simulink model "Kalman_Filter_Simulink_Example_adap_SMNSF"  (R2018a)
settings: Solver=FixedStepAuto  StartTime=0.0  StopTime=40  FixedStep=.01  RelTol=1e-3
values from neighbouring files (symbols this model uses):
  g = 9.81    [Kalman_Filter_Simulink_Example_params_EKF.m]
  l = 0.5    [Kalman_Filter_Simulink_Example_params_EKF.m]
  P0 = [10 0; 0 10]    [Kalman_Filter_Simulink_Example_params_EKF.m]
  Q = 1e-4    (= 0.0001)    [Kalman_Filter_Simulink_Example_params_EKF.m]
  Q0 = 2e-4    (= 0.0002)    [Kalman_Filter_Simulink_Example_params_EKF.m]
  R = 1e-3    (= 0.001)    [Kalman_Filter_Simulink_Example_params_EKF.m]
  R0 = 2e-3    (= 0.002)    [Kalman_Filter_Simulink_Example_params_EKF.m]
  theta0 = pi/4    (= 0.785398163397)    [Kalman_Filter_Simulink_Example_params_EKF.m]
  Ts = 0.01    [Kalman_Filter_Simulink_Example_params_EKF.m]
libraries: Bias x9, simulink x4, sharedTrackingLibrary x1, Meldas_Library x1
settings Model: Creator=mulusoy  LastModifiedBy=hussein
settings OptimizationCC: DefaultParameterBehavior=Inlined  PassReuseOutputArgsAs=Individual arguments
settings DebuggingCC: ParameterTunabilityLossMsg=error
settings SFSimCC: MATLABDynamicMemAlloc=off
settings RTWCC: SystemTargetFile=ert.tlc  TemplateMakefile=ert_default_tmf  GenerateReport=on  IncludeHyperlinkInReport=on  LaunchReport=on  GenerateTraceInfo=on  GenerateTraceReport=on  GenerateTraceReportSl=on  GenerateTraceReportSf=on  GenerateTraceReportEml=on  CheckMdlBeforeBuild=Warning
settings CodeAppCC: GenerateComments=off  IgnoreCustomStorageClasses=off  SimulinkBlockComments=off
settings ERTTargetCC: TargetLangStandard=C99 (ISO)  GenerateSampleERTMain=on  InlinedParameterPlacement=NonHierarchical  ERTCustomFileTemplate=example_file_process.tlc
settings SimscapeCC: SimscapeNormalizeSystem=off

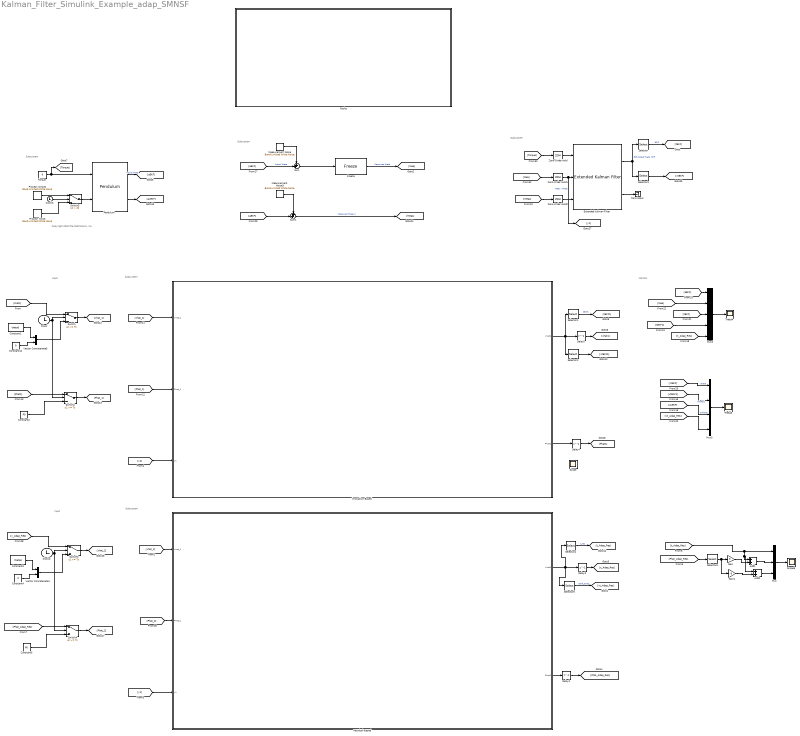
== system Kalman_Filter_Simulink_Example_adap_SMNSF ==
  note: Subsystem
  note: Subsystem
  note: Monitor
  note: Input
  note: Input
  note: Subsystem
  note: Subsystem
  note: Copyright 2018 The MathWorks, Inc.
  note: Subsystem
  Add1 : Sum
  Add2 : Sum
  Clock : Clock
      settings: Decimation=1000
  Clock2 : Clock
      settings: Decimation=1000
  Clock3 : Clock
  Constant1 : Constant  Value=theta0
  Constant12 : Constant  Value=0
  Constant2 : Constant  Value=P0
  Constant3 : Constant  Value=theta0
  Constant4 : Constant  Value=0
  Constant5 : Constant  Value=P0
  Delay{2..5} (4 alike) : Delay  DelayLength=1
  Extended Kalman Filter : sharedTrackingLibrary/Extended Kalman Filter  StateTransitionFcn=myStateTransitionFcn  HasStateTransitionJacobianFcn=off  HasAdditiveProcessNoise=Additive  ProcessNoise=diag([0,Q0])  HasTimeVaryingProcessNoise=off  HasStateTransitionFcnExtraArgument=1  InitialState=[pi/4 0]  InitialStateCovariance=10  MeasurementFcn1=myMeasurementFcn  HasMeasurementJacobianFcn1=off  HasMeasurementEnablePort1=off  HasAdditiveMeasurementNoise1=Additive  MeasurementNoise1=R0  HasTimeVaryingMeasurementNoise1=off  HasMeasurementFcnExtraArgument1=0  MeasurementFcn2=myMeasurementFcn  HasMeasurementJacobianFcn2=off  HasMeasurementEnablePort2=off  HasAdditiveMeasurementNoise2=Additive  MeasurementNoise2=R0  HasTimeVaryingMeasurementNoise2=off  HasMeasurementFcnExtraArgument2=0  MeasurementFcn3=myMeasurementFcn  HasMeasurementJacobianFcn3=off  HasMeasurementEnablePort3=off  HasAdditiveMeasurementNoise3=Additive  MeasurementNoise3=1  HasTimeVaryingMeasurementNoise3=off  HasMeasurementFcnExtraArgument3=0  MeasurementFcn4=myMeasurementFcn  HasMeasurementJacobianFcn4=off  HasMeasurementEnablePort4=off  HasAdditiveMeasurementNoise4=Additive  MeasurementNoise4=1  HasTimeVaryingMeasurementNoise4=off  HasMeasurementFcnExtraArgument4=0  MeasurementFcn5=myMeasurementFcn  HasMeasurementJacobianFcn5=off  HasMeasurementEnablePort5=off  HasAdditiveMeasurementNoise5=Additive  MeasurementNoise5=1  HasTimeVaryingMeasurementNoise5=off  HasMeasurementFcnExtraArgument5=0  EnableMultirate=off  StateTransitionFcnSampleTime=1  MeasurementFcn1SampleTime=1  MeasurementFcn2SampleTime=1  MeasurementFcn3SampleTime=1  MeasurementFcn4SampleTime=1  MeasurementFcn5SampleTime=1  UseCurrentEstimator=on  OutputStateCovariance=on  DataType=double  SampleTime=Ts  NumberOfMeasurements=2
      settings: SourceProductName=Control System Toolbox  SourceProductBaseCode=CT
  Faults : Subsystem
  Freeze : Bias/Freeze  Time=5
  Gain : Gain  Gain=3
  Gain1 : Gain  Gain=-3
  Innovation-Based : Subsystem
  Measurement Noise : simulink/Sources/Band-Limited White Noise  Cov=R*Ts  Ts=Ts  seed=[12347]
  Measurement Noise3 : simulink/Sources/Band-Limited White Noise  Cov=R*Ts  Ts=Ts  seed=[12347]
  Mux : Mux  Inputs=3
  Mux2 : Mux  Inputs=5
  Mux3 : Mux
  Pendulum : Meldas_Library/Pendulum  theta_0=pi/3  theta_dot_0=0
  Process Noise2 : simulink/Sources/Band-Limited White Noise  Cov=Q*Ts*1000  Ts=Ts  seed=[12347]
  Process Noise : simulink/Sources/Band-Limited White Noise  Cov=0  Ts=Ts  seed=[23341]
  Residual-Based : Subsystem
  Scope5 : Scope
  Selector : Selector  InputPortWidth=2  IndexOptions=Index vector (dialog)  Indices=1  OutputSizes=1
  Selector1 : Selector  InputPortWidth=2  IndexOptions=Index vector (dialog)  Indices=1  OutputSizes=1
  Selector2 : Selector  InputPortWidth=2  IndexOptions=Index vector (dialog)  Indices=2  OutputSizes=1
  Selector3 : Selector  InputPortWidth=2  IndexOptions=Index vector (dialog)  Indices=2  OutputSizes=1
  Selector4 : Selector  InputPortWidth=2  IndexOptions=Index vector (dialog)  Indices=1  OutputSizes=1
  Selector5 : Selector  InputPortWidth=2  IndexOptions=Index vector (dialog)  Indices=2  OutputSizes=1
  Selector6 : Selector  NumberOfDimensions=2  InputPortWidth=3  IndexOptions=Index vector (dialog),Index vector (dialog)  Indices=1,1  OutputSizes=1,1
  Sum : Sum  Inputs=++|
  Sum1 : Sum  Inputs=++|
  Switch{,1,3..4} (4 alike) : Switch  Threshold=Ts
  Switch5 : Switch  Criteria=u2 > Threshold  Threshold=40
  Terminator : Terminator
  Theta4 : Scope
  Theta5 : Scope
  Torque : Constant  Value=0
  Vector Concatenate1 : Concatenate
  Vector Concatenate5 : Concatenate
  Zero-Order Hold : ZeroOrderHold  SampleTime=Ts
  Zero-Order Hold1 : ZeroOrderHold  SampleTime=Ts
  Zero-Order Hold2 : ZeroOrderHold  SampleTime=Ts
  Scope : Scope
  wires:
  Clock/1 -> Switch1/2, Switch/2
  Constant1/1 -> Vector Concatenate5/1
  Constant2/1 -> Switch1/3
  Constant12/1 -> Vector Concatenate5/2
  Vector Concatenate5/1 -> Switch/3
  [xhat1] -> Switch/1
  [Phat1] -> Switch1/1
  Switch/1 -> [xhat_1]
  Switch1/1 -> [Phat_1]
  [Phat_1] -> Innovation-Based/2(Phat_1)
  [y1] -> Innovation-Based/3(y1)
  Innovation-Based/2(Phat1) -> Delay4/1
  Selector2/1 -> [vtEKF1]
  Innovation-Based/1(xhat1) -> Selector2/1, Selector1/1, Delay5/1
  Selector1/1 -> [tEKF1]  "tEKF1"
  [xhat_1] -> Innovation-Based/1(xhat_1)
  Residual-Based/2(Phat1) -> Delay2/1
  Residual-Based/1(xhat1) -> Selector5/1, Selector4/1, Delay3/1
  Selector5/1 -> [vt_Adap_Res]  "vEKF_adap"
  [y1] -> Residual-Based/3(y1)
  Clock2/1 -> Switch4/2, Switch3/2
  Switch4/1 -> [Phat_2]
  Constant5/1 -> Switch4/3
  Vector Concatenate1/1 -> Switch3/3
  Constant3/1 -> Vector Concatenate1/1
  Switch3/1 -> [xhat_2]
  [Phat_Adap_Res] -> Switch4/1
  Constant4/1 -> Vector Concatenate1/2
  [x_Adap_Res] -> Switch3/1
  [xhat_2] -> Residual-Based/1(xhat_1)
  [Phat_2] -> Residual-Based/2(Phat_1)
  [Mea] -> Mux2/2
  [vtEKF] -> Mux3/1  "vtheta"
  Mux3/1 -> Theta5/1
  [tEKF1] -> Mux2/4
  Mux2/1 -> Theta4/1
  [vtEKF1] -> Mux3/2  "vtheta1"
  [avEKF] -> Mux3/3  "aVtheta"
  [tEKF] -> Mux2/3
  [aEKF] -> Mux2/1
  [vt_Adap_Res] -> Mux3/4
  [t_Adap_Res] -> Mux2/5
  [Phat_Adap_Res] -> Selector6/1
  [t_Adap_Res] -> Add2/1, Add1/1, Mux/1
  Selector6/1 -> Gain1/1, Gain/1
  Gain/1 -> Add1/2
  Add1/1 -> Mux/2
  Gain1/1 -> Add2/2
  Add2/1 -> Mux/3
  Mux/1 -> Scope5/1
  Selector4/1 -> [t_Adap_Res]  "t_res"
  Delay2/1 -> [Phat_Adap_Res]
  Delay3/1 -> [x_Adap_Res]
  Delay4/1 -> [Phat1]
  Delay5/1 -> [xhat1]
  Pendulum/1 -> [aEKF]  "Actual theta"
  Pendulum/2 -> [avEKF]
  [aEKF] -> Sum1/2
  Sum/1 -> Freeze/1
  Process Noise/1 -> Switch5/3
  Measurement Noise/1 -> Sum/1
  [aEKF] -> Sum/2  "Actual theta"
  Clock3/1 -> Switch5/2
  Torque/1 -> Pendulum/1, [Torque]
  Measurement Noise3/1 -> Sum1/1
  Freeze/1 -> [Mea]  "Measured theta"
  Process Noise2/1 -> Switch5/1
  Sum1/1 -> [Mea1]  "Measured theta 2"
  Switch5/1 -> Pendulum/2
  Zero-Order Hold1/1 -> [y1], Extended Kalman Filter/2  "Meas  Theta"
  Extended Kalman Filter/1 -> Selector3/1, Selector/1  "Estimated theta  EKF"
  Zero-Order Hold/1 -> Extended Kalman Filter/1
  Selector/1 -> [tEKF]  "tEKF"
  Selector3/1 -> [vtEKF]
  [Mea] -> Zero-Order Hold1/1
  [Mea1] -> Zero-Order Hold2/1
  Zero-Order Hold2/1 -> Extended Kalman Filter/3
  [Torque] -> Zero-Order Hold/1
  Extended Kalman Filter/2 -> Terminator/1

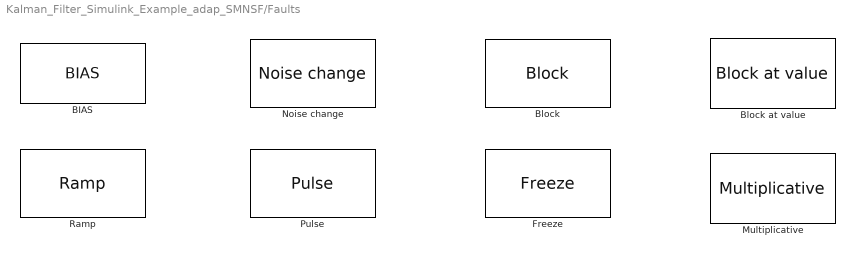
== system Kalman_Filter_Simulink_Example_adap_SMNSF/Faults ==
  BIAS : Bias/BIAS  Bias=0  Time=0
  Block : Bias/Block  Noise=0  Time=0
  Block at value : Bias/Block at value  Value=0  Time=0
  Freeze : Bias/Freeze  Time=0
  Multiplicative : Bias/Multiplicative  Gain=0  Time=0
  Noise change : Bias/Noise change  Noise_add=0  Time=0
  Pulse : Bias/Pulse  Pulse_value=0.1  Pulse_periode=0  Pulse_width=0  Time=0
  Ramp : Bias/Ramp  Slope=0  Time=0

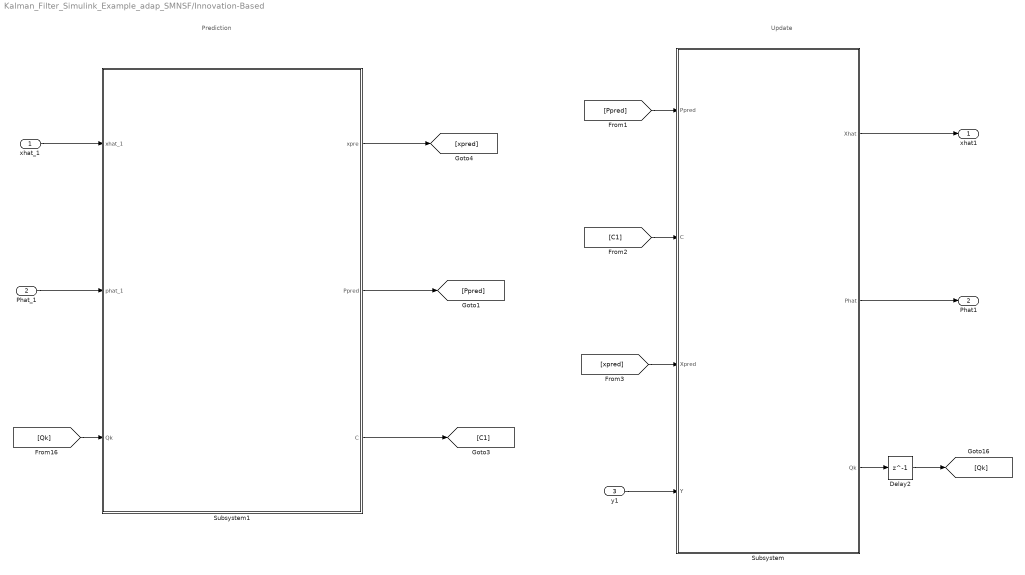
== system Kalman_Filter_Simulink_Example_adap_SMNSF/Innovation-Based ==
  note: Update
  note: Prediction
  xhat_1 : Inport
  Phat_1 : Inport  Port=2
  y1 : Inport  Port=3
  Delay2 : Delay  DelayLength=1  SampleTime=Ts
  Subsystem : Subsystem
  Subsystem1 : Subsystem
  xhat1 : Outport
  Phat1 : Outport  Port=2
  wires:
  [Ppred] -> Subsystem/1(Ppred)
  Subsystem/3(Qk) -> Delay2/1
  y1/1 -> Subsystem/4("Y ")
  Delay2/1 -> [Qk]
  Subsystem/2("Phat ") -> Phat1/1
  Subsystem1/1(xpre) -> [xpred]
  [C1] -> Subsystem/2(C)
  Phat_1/1 -> Subsystem1/2("phat_1 ")
  [xpred] -> Subsystem/3(Xpred)
  xhat_1/1 -> Subsystem1/1(xhat_1)
  Subsystem1/2(Ppred) -> [Ppred]
  Subsystem1/3("C ") -> [C1]
  Subsystem/1(Xhat) -> xhat1/1
  [Qk] -> Subsystem1/3("Qk ")

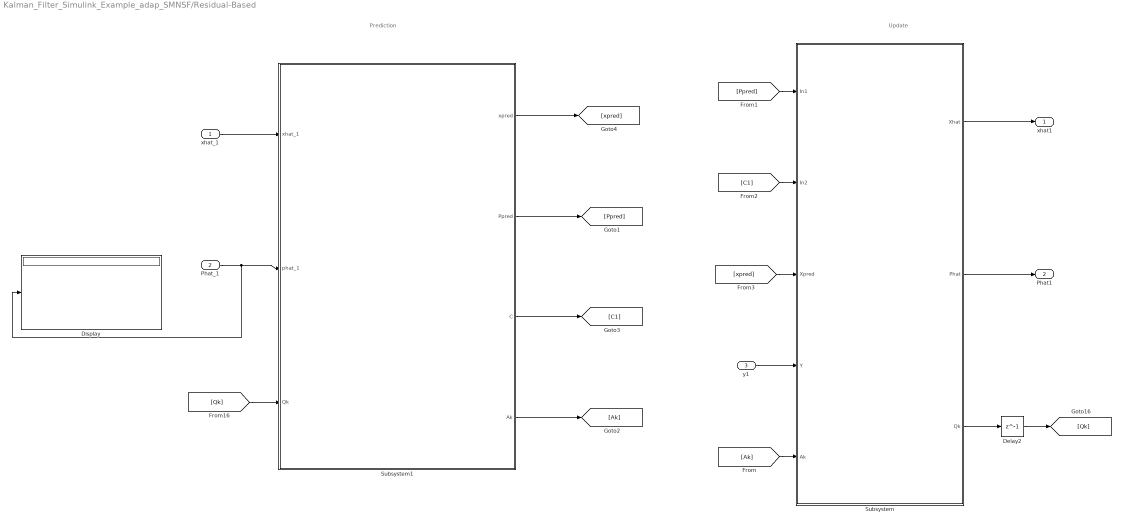
== system Kalman_Filter_Simulink_Example_adap_SMNSF/Residual-Based ==
  note: Update
  note: Prediction
  xhat_1 : Inport
  Phat_1 : Inport  Port=2
  y1 : Inport  Port=3
  Delay2 : Delay  DelayLength=1  SampleTime=Ts
  Display : Display
  Subsystem : Subsystem
  Subsystem1 : Subsystem
  xhat1 : Outport
  Phat1 : Outport  Port=2
  wires:
  [Ppred] -> Subsystem/1(In1)
  y1/1 -> Subsystem/4("Y ")
  Delay2/1 -> [Qk]
  Subsystem/2("Phat ") -> Phat1/1
  Subsystem1/1(xpred) -> [xpred]
  [C1] -> Subsystem/2(In2)
  Phat_1/1 -> Display/1, Subsystem1/2(phat_1)
  [xpred] -> Subsystem/3(Xpred)
  xhat_1/1 -> Subsystem1/1(xhat_1)
  Subsystem1/2(Ppred) -> [Ppred]
  Subsystem1/3("C ") -> [C1]
  Subsystem/1(Xhat) -> xhat1/1
  [Qk] -> Subsystem1/3("Qk ")
  Subsystem1/4(Ak) -> [Ak]
  [Ak] -> Subsystem/5("Ak ")
  Subsystem/3(Qk) -> Delay2/1

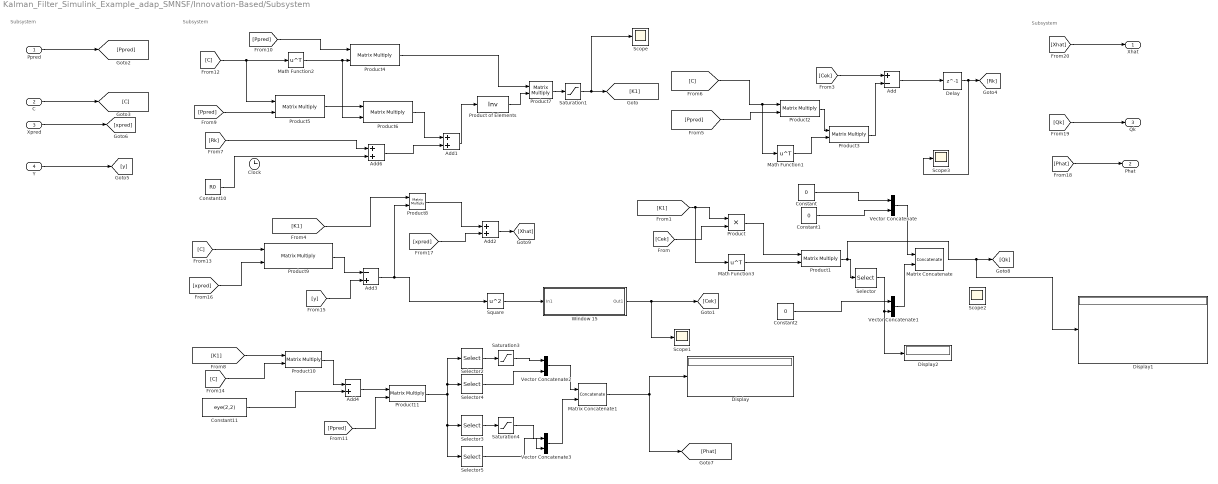
== system Kalman_Filter_Simulink_Example_adap_SMNSF/Innovation-Based/Subsystem ==
  note: Subsystem
  note: Subsystem
  note: Subsystem
  Ppred : Inport
  C : Inport  Port=2
  Xpred : Inport  Port=3
  "Y " : Inport  Port=4
  Add : Sum  Inputs=+-
  Add1 : Sum
  Add2 : Sum
  Add3 : Sum  Inputs=-+
  Add4 : Sum  Inputs=-+
  Add6 : Sum
  Clock : Clock
  Constant : Constant  Value=0
  Constant1 : Constant  Value=0
  Constant10 : Constant  Value=R0
  Constant11 : Constant  Value=eye(2,2)
  Constant2 : Constant  Value=0
  Delay : Delay  DelayLength=1
  Display : Display
  Display1 : Display
  Display2 : Display
  Math Function1 : Math  Operator=transpose  SaturateOnIntegerOverflow=on
  Math Function2 : Math  Operator=transpose  SaturateOnIntegerOverflow=on
  Math Function3 : Math  Operator=transpose  SaturateOnIntegerOverflow=on
  Matrix Concatenate : Concatenate  Mode=Multidimensional array  ConcatenateDimension=2
  Matrix Concatenate1 : Concatenate  Mode=Multidimensional array  ConcatenateDimension=2
  Product : Product
  Product of Elements : Product  Inputs=/  Multiplication=Matrix(*)
  Product{1..11} (11 alike) : Product  Multiplication=Matrix(*)
  Saturation1 : Saturate  UpperLimit=1  LowerLimit=0
  Saturation3 : Saturate  UpperLimit=1  LowerLimit=0
  Saturation4 : Saturate  UpperLimit=1  LowerLimit=0
  Scope{,1..3} (4 alike) : Scope
  Selector : Selector  NumberOfDimensions=2  InputPortWidth=3  IndexOptions=Index vector (dialog),Index vector (dialog)  Indices=2,2  OutputSizes=1,1
  Selector2 : Selector  NumberOfDimensions=2  InputPortWidth=3  IndexOptions=Index vector (dialog),Index vector (dialog)  Indices=1,1  OutputSizes=1,1
  Selector3 : Selector  NumberOfDimensions=2  InputPortWidth=3  IndexOptions=Index vector (dialog),Index vector (dialog)  Indices=2,2  OutputSizes=1,1
  Selector4 : Selector  NumberOfDimensions=2  InputPortWidth=3  IndexOptions=Index vector (dialog),Index vector (dialog)  Indices=2,1  OutputSizes=1,1
  Selector5 : Selector  NumberOfDimensions=2  InputPortWidth=3  IndexOptions=Index vector (dialog),Index vector (dialog)  Indices=1,2  OutputSizes=1,1
  Square : Math  Operator=square  SaturateOnIntegerOverflow=on
  Vector Concatenate{,1..3} (4 alike) : Concatenate
  Window 15 : Subsystem
  Xhat : Outport  PortDimensions=[2,1]
  "Phat " : Outport  Port=2  PortDimensions=[2,2]
  Qk : Outport  Port=3  PortDimensions=[2,2]
  wires:
  Ppred/1 -> [Ppred]
  C/1 -> [C]
  Xpred/1 -> [xpred]
  "Y "/1 -> [y]
  [Xhat] -> Xhat/1
  [Phat] -> "Phat "/1
  [Qk] -> Qk/1
  Product2/1 -> Product3/1
  [xpred] -> Add2/2
  Add4/1 -> Product11/1
  [Ppred] -> Product2/2
  [K1] -> Product10/1
  [xpred] -> Product9/2
  [K1] -> Product8/1
  Math Function1/1 -> Product3/2
  Square/1 -> Window 15/1(In1)
  [K1] -> Math Function3/1, Product/1
  [Cek] -> Add/1
  [Cek] -> Product/2
  Math Function2/1 -> Product6/2, Product4/2
  Product of Elements/1 -> Product7/2
  Add1/1 -> Product of Elements/1
  Product8/1 -> Add2/1
  Product3/1 -> Add/2
  Product/1 -> Product1/1
  [Rk] -> Add6/1
  Constant11/1 -> Add4/2
  [Ppred] -> Product11/2
  [y] -> Add3/2
  [C] -> Math Function1/1, Product2/1
  Product10/1 -> Add4/1
  Product6/1 -> Add1/1
  [C] -> Product9/1
  Add3/1 -> Square/1, Product8/2
  Add2/1 -> [Xhat]
  Product4/1 -> Product7/1
  Product5/1 -> Product6/1
  [C] -> Product10/2
  [Ppred] -> Product4/1
  Product9/1 -> Add3/1
  [Ppred] -> Product5/2
  [C] -> Product5/1, Math Function2/1
  Product1/1 -> Display1/1, [Qk], Selector/1
  Constant/1 -> Vector Concatenate/1
  Constant1/1 -> Vector Concatenate/2
  Constant2/1 -> Vector Concatenate1/1
  Vector Concatenate/1 -> Matrix Concatenate/1
  Math Function3/1 -> Product1/2
  Window 15/1(Out1) -> Scope1/1, [Cek]
  Add/1 -> Delay/1
  Vector Concatenate1/1 -> Matrix Concatenate/2
  Selector/1 -> Display2/1, Vector Concatenate1/2
  Constant10/1 -> Add6/2
  Add6/1 -> Add1/2
  Product7/1 -> Saturation1/1
  Delay/1 -> Scope3/1, [Rk]
  Saturation1/1 -> Scope/1, [K1]
  Vector Concatenate2/1 -> Matrix Concatenate1/1
  Matrix Concatenate1/1 -> Display/1, [Phat]
  Selector4/1 -> Vector Concatenate2/2
  Vector Concatenate3/1 -> Matrix Concatenate1/2
  Selector3/1 -> Saturation4/1
  Selector5/1 -> Vector Concatenate3/1
  Saturation3/1 -> Vector Concatenate2/1
  Product11/1 -> Selector5/1, Selector3/1, Selector4/1, Selector2/1
  Saturation4/1 -> Vector Concatenate3/2
  Selector2/1 -> Saturation3/1

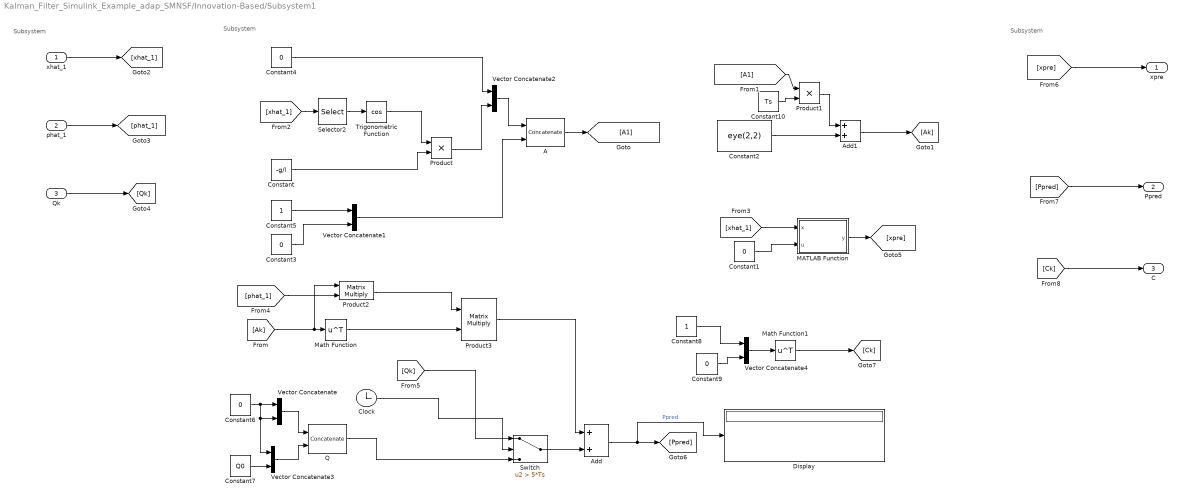
== system Kalman_Filter_Simulink_Example_adap_SMNSF/Innovation-Based/Subsystem1 ==
  note: Subsystem
  note: Subsystem
  note: Subsystem
  xhat_1 : Inport
  "phat_1 " : Inport  Port=2
  "Qk " : Inport  Port=3
  A : Concatenate  Mode=Multidimensional array  ConcatenateDimension=2
  Add : Sum
  Add1 : Sum
  Clock : Clock
      settings: Decimation=1000
  Constant : Constant  Value=-g/l
  Constant{1,3..4,6,9} (5 alike) : Constant  Value=0
  Constant10 : Constant  Value=Ts
  Constant2 : Constant  Value=eye(2,2)
  Constant5 : Constant
  Constant7 : Constant  Value=Q0
  Constant8 : Constant
  Display : Display
  MATLAB Function : MATLAB Function  TreatAsAtomicUnit=on
  Math Function : Math  Operator=transpose  SaturateOnIntegerOverflow=on
  Math Function1 : Math  Operator=transpose  SaturateOnIntegerOverflow=on
  Product : Product
  Product1 : Product
  Product2 : Product  Multiplication=Matrix(*)
  Product3 : Product  Multiplication=Matrix(*)
  Q : Concatenate  Mode=Multidimensional array  ConcatenateDimension=2
  Selector2 : Selector  InputPortWidth=2  IndexOptions=Index vector (dialog)  Indices=1  OutputSizes=1
  Switch : Switch  Criteria=u2 > Threshold  Threshold=5*Ts
  Trigonometric Function : Trigonometry  Operator=cos
  Vector Concatenate{,1..4} (5 alike) : Concatenate
  xpre : Outport
  Ppred : Outport  Port=2
  "C " : Outport  Port=3
  wires:
  "Qk "/1 -> [Qk]
  xhat_1/1 -> [xhat_1]
  "phat_1 "/1 -> [phat_1]
  [xpre] -> xpre/1
  [Ppred] -> Ppred/1
  [Ck] -> "C "/1
  Constant10/1 -> Product1/2
  [A1] -> Product1/1
  Constant/1 -> Product/2
  [xhat_1] -> MATLAB Function/1(x)
  Selector2/1 -> Trigonometric Function/1
  Constant9/1 -> Vector Concatenate4/2
  Vector Concatenate2/1 -> A/1
  Product/1 -> Vector Concatenate2/2
  Constant5/1 -> Vector Concatenate1/1
  A/1 -> [A1]
  Vector Concatenate1/1 -> A/2
  Math Function/1 -> Product3/2
  Product3/1 -> Add/1
  Constant3/1 -> Vector Concatenate1/2
  Product2/1 -> Product3/1
  Vector Concatenate4/1 -> Math Function1/1
  Product1/1 -> Add1/1
  Constant1/1 -> MATLAB Function/2(u)
  Constant7/1 -> Vector Concatenate3/2
  Vector Concatenate3/1 -> Q/2
  [Ak] -> Math Function/1, Product2/1
  Constant8/1 -> Vector Concatenate4/1
  Trigonometric Function/1 -> Product/1
  Add/1 -> Display/1, [Ppred]  "Ppred"
  [xhat_1] -> Selector2/1
  Constant2/1 -> Add1/2
  [phat_1] -> Product2/2
  MATLAB Function/1(y) -> [xpre]
  Clock/1 -> Switch/2
  Add1/1 -> [Ak]
  Math Function1/1 -> [Ck]
  Vector Concatenate/1 -> Q/1
  Constant4/1 -> Vector Concatenate2/1
  Q/1 -> Switch/3
  Constant6/1 -> Vector Concatenate3/1, Vector Concatenate/2, Vector Concatenate/1
  Switch/1 -> Add/2
  [Qk] -> Switch/1

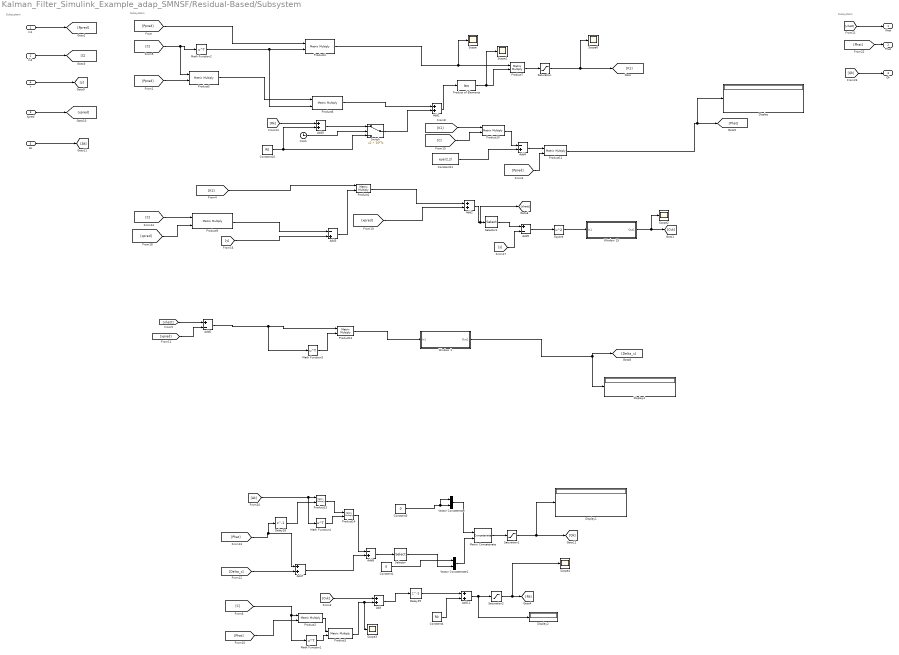
== system Kalman_Filter_Simulink_Example_adap_SMNSF/Residual-Based/Subsystem ==
  note: Subsystem
  note: Subsystem
  note: Subsystem
  In1 : Inport
  In2 : Inport  Port=2
  Xpred : Inport  Port=3
  "Y " : Inport  Port=4
  "Ak " : Inport  Port=5
  Add{,1..2,7,9,11} (6 alike) : Sum
  Add3 : Sum  Inputs=-+
  Add4 : Sum  Inputs=-+
  Add5 : Sum  Inputs=+-
  Add6 : Sum  Inputs=+-
  Add8 : Sum  Inputs=-+
  Clock : Clock
  Constant1 : Constant  Value=0
  Constant10 : Constant  Value=R0
  Constant11 : Constant  Value=eye(2,2)
  Constant3 : Constant  Value=0
  Constant4 : Constant  Value=R0
  Delay28 : Delay  DelayLength=1
  Delay29 : Delay  DelayLength=1
  Display{,1..2,4} (4 alike) : Display
  Math Function{1..4} (4 alike) : Math  Operator=transpose  SaturateOnIntegerOverflow=on
  Matrix Concatenate : Concatenate  Mode=Multidimensional array  ConcatenateDimension=2
  Product of Elements : Product  Inputs=/  Multiplication=Matrix(*)
  Product{1..7,9..14} (13 alike) : Product  Multiplication=Matrix(*)
  Saturation : Saturate  UpperLimit=1  LowerLimit=0
  Saturation1 : Saturate  UpperLimit=1  LowerLimit=0
  Saturation2 : Saturate  UpperLimit=1  LowerLimit=0
  Scope{,1..4,6} (6 alike) : Scope
  Selector : Selector  NumberOfDimensions=2  InputPortWidth=3  IndexOptions=Index vector (dialog),Index vector (dialog)  Indices=2,2  OutputSizes=1,1
  Selector1 : Selector  InputPortWidth=2  IndexOptions=Index vector (dialog)  Indices=1  OutputSizes=1
  Square : Math  Operator=square  SaturateOnIntegerOverflow=on
  Switch : Switch  Criteria=u2 > Threshold  Threshold=20*Ts
  Vector Concatenate : Concatenate
  Vector Concatenate1 : Concatenate
  Window 1 : Subsystem
  Window 15 : Subsystem
  Xhat : Outport  PortDimensions=[2,1]
  "Phat " : Outport  Port=2
  Qk : Outport  Port=3  PortDimensions=[2,2]
  wires:
  Add2/1 -> [xhatt], Selector1/1
  Add5/1 -> Square/1
  [K1] -> Product1/1
  [Ppred] -> Product4/1
  Add3/1 -> Product1/2
  Product of Elements/1 -> Scope1/1, Product7/2
  Product5/1 -> Product6/1
  Product9/1 -> Add3/1
  Math Function2/1 -> Product6/2, Product4/2
  [xhatt] -> Add6/1
  Add1/1 -> Product of Elements/1
  Window 1/1(Out1) -> [Delta_x], Display4/1
  [xpred] -> Add6/2
  Math Function3/1 -> Product12/2
  Product6/1 -> Add1/1
  Selector1/1 -> Add5/1
  Product1/1 -> Add2/1
  [Ppred] -> Product5/2
  Add6/1 -> Product12/1, Math Function3/1
  [C] -> Product9/1
  Window 15/1(Out1) -> Scope2/1, [Cvk]
  [C] -> Product5/1, Math Function2/1
  [y] -> Add3/2
  [y] -> Add5/2
  [xpred] -> Product9/2
  [xpred] -> Add2/2
  "Y "/1 -> [y]
  In1/1 -> [Ppred]
  In2/1 -> [C]
  "Ak "/1 -> [Ak]
  Xpred/1 -> [xpred]
  [xhatt] -> Xhat/1
  [Phat] -> "Phat "/1
  [Qk] -> Qk/1
  Add4/1 -> Product11/1
  [C] -> Product10/2
  Product10/1 -> Add4/1
  [Ppred] -> Product11/2
  [K1] -> Product10/1
  Constant11/1 -> Add4/2
  [Delta_x] -> Add7/2
  [Cvk] -> Add/1
  Math Function1/1 -> Product3/2
  Product13/1 -> Product14/1
  [C] -> Math Function1/1, Product2/1
  Product14/1 -> Add8/1
  Product2/1 -> Product3/1
  [Phat] -> Delay28/1, Add7/1
  Math Function4/1 -> Product14/2
  Add7/1 -> Add8/2
  Product3/1 -> Add/2, Scope3/1
  Vector Concatenate1/1 -> Matrix Concatenate/2
  Constant1/1 -> Vector Concatenate1/1
  Vector Concatenate/1 -> Matrix Concatenate/1
  Constant3/1 -> Vector Concatenate/1, Vector Concatenate/2
  Add8/1 -> Selector/1
  Delay28/1 -> Product13/2
  Add/1 -> Delay29/1
  Product4/1 -> Scope/1, Product7/1
  Product7/1 -> Saturation/1
  [Phat] -> Product2/2
  Delay29/1 -> Add11/1
  Constant4/1 -> Add11/2
  Add11/1 -> Display2/1, Saturation2/1
  Matrix Concatenate/1 -> Saturation1/1
  Selector/1 -> Vector Concatenate1/2
  [Ak] -> Math Function4/1, Product13/1
  Saturation/1 -> Scope6/1, [K1]
  Square/1 -> Window 15/1(In1)
  Switch/1 -> Add1/2
  [Rk] -> Add9/1
  Clock/1 -> Switch/2
  Constant10/1 -> Add9/2, Switch/3
  Saturation1/1 -> [Qk], Display1/1
  Saturation2/1 -> Scope4/1, [Rk]
  Product11/1 -> Display/1, [Phat]
  Product12/1 -> Window 1/1(In1)
  Add9/1 -> Switch/1

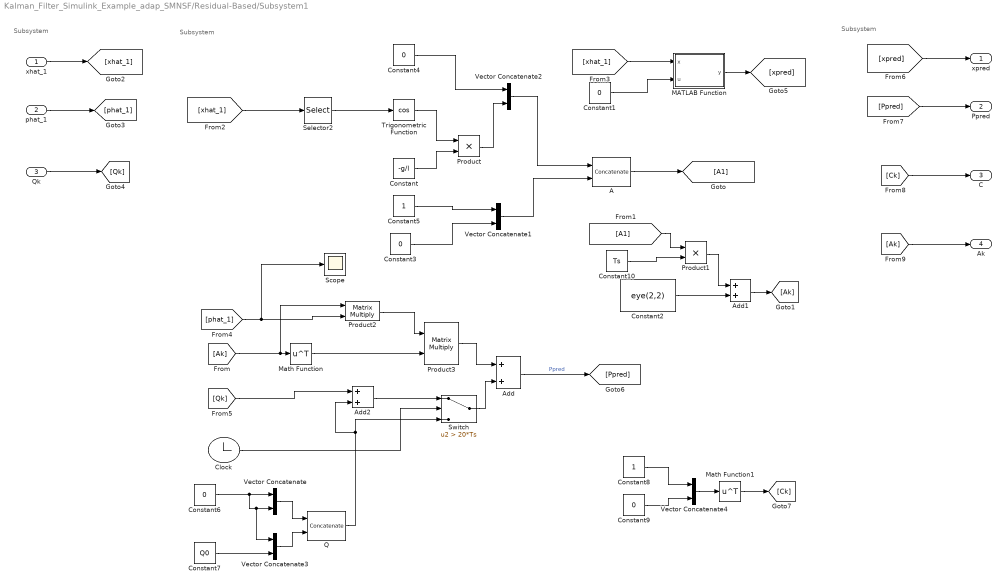
== system Kalman_Filter_Simulink_Example_adap_SMNSF/Residual-Based/Subsystem1 ==
  note: Subsystem
  note: Subsystem
  note: Subsystem
  xhat_1 : Inport
  phat_1 : Inport  Port=2
  "Qk " : Inport  Port=3
  A : Concatenate  Mode=Multidimensional array  ConcatenateDimension=2
  Add : Sum
  Add1 : Sum
  Add2 : Sum
  Clock : Clock
      settings: Decimation=1000
  Constant : Constant  Value=-g/l
  Constant{1,3..4,6,9} (5 alike) : Constant  Value=0
  Constant10 : Constant  Value=Ts
  Constant2 : Constant  Value=eye(2,2)
  Constant5 : Constant
  Constant7 : Constant  Value=Q0
  Constant8 : Constant
  MATLAB Function : MATLAB Function  TreatAsAtomicUnit=on
  Math Function : Math  Operator=transpose  SaturateOnIntegerOverflow=on
  Math Function1 : Math  Operator=transpose  SaturateOnIntegerOverflow=on
  Product : Product
  Product1 : Product
  Product2 : Product  Multiplication=Matrix(*)
  Product3 : Product  Multiplication=Matrix(*)
  Q : Concatenate  Mode=Multidimensional array  ConcatenateDimension=2
  Scope : Scope
  Selector2 : Selector  InputPortWidth=2  IndexOptions=Index vector (dialog)  Indices=1  OutputSizes=1
  Switch : Switch  Criteria=u2 > Threshold  Threshold=20*Ts
  Trigonometric Function : Trigonometry  Operator=cos
  Vector Concatenate{,1..4} (5 alike) : Concatenate
  xpred : Outport
  Ppred : Outport  Port=2
  "C " : Outport  Port=3
  Ak : Outport  Port=4
  wires:
  phat_1/1 -> [phat_1]
  xhat_1/1 -> [xhat_1]
  "Qk "/1 -> [Qk]
  [xpred] -> xpred/1
  [Ppred] -> Ppred/1
  [Ck] -> "C "/1
  [Ak] -> Ak/1
  Add1/1 -> [Ak]
  Constant2/1 -> Add1/2
  [A1] -> Product1/1
  [xhat_1] -> Selector2/1
  A/1 -> [A1]
  Constant4/1 -> Vector Concatenate2/1
  Constant9/1 -> Vector Concatenate4/2
  Vector Concatenate2/1 -> A/1
  Vector Concatenate4/1 -> Math Function1/1
  Trigonometric Function/1 -> Product/1
  [phat_1] -> Scope/1, Product2/2
  Product2/1 -> Product3/1
  Constant10/1 -> Product1/2
  [Ak] -> Product2/1, Math Function/1
  Product/1 -> Vector Concatenate2/2
  Selector2/1 -> Trigonometric Function/1
  Vector Concatenate3/1 -> Q/2
  Vector Concatenate1/1 -> A/2
  Product1/1 -> Add1/1
  Math Function/1 -> Product3/2
  Vector Concatenate/1 -> Q/1
  Constant6/1 -> Vector Concatenate3/1, Vector Concatenate/2, Vector Concatenate/1
  Constant1/1 -> MATLAB Function/2(u)
  Constant5/1 -> Vector Concatenate1/1
  Constant3/1 -> Vector Concatenate1/2
  Constant/1 -> Product/2
  Math Function1/1 -> [Ck]
  Product3/1 -> Add/1
  MATLAB Function/1(y) -> [xpred]
  [xhat_1] -> MATLAB Function/1(x)
  Constant8/1 -> Vector Concatenate4/1
  Constant7/1 -> Vector Concatenate3/2
  Add/1 -> [Ppred]  "Ppred"
  Clock/1 -> Switch/2
  Switch/1 -> Add/2
  [Qk] -> Add2/1
  Q/1 -> Add2/2, Switch/3
  Add2/1 -> Switch/1

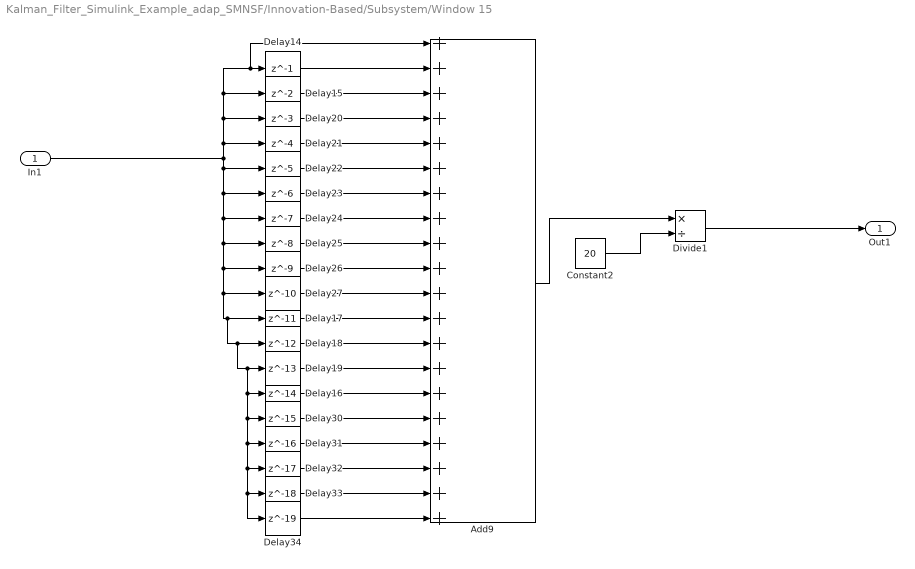
== system Kalman_Filter_Simulink_Example_adap_SMNSF/Innovation-Based/Subsystem/Window 15 ==
  In1 : Inport
  Add9 : Sum  Inputs=20
  Constant2 : Constant  Value=20
  Delay14 : Delay  DelayLength=1  SampleTime=Ts
  Delay15 : Delay  SampleTime=Ts
  Delay16 : Delay  DelayLength=14  SampleTime=Ts
  Delay17 : Delay  DelayLength=11  SampleTime=Ts
  Delay18 : Delay  DelayLength=12  SampleTime=Ts
  Delay19 : Delay  DelayLength=13  SampleTime=Ts
  Delay20 : Delay  DelayLength=3  SampleTime=Ts
  Delay21 : Delay  DelayLength=4  SampleTime=Ts
  Delay22 : Delay  DelayLength=5  SampleTime=Ts
  Delay23 : Delay  DelayLength=6  SampleTime=Ts
  Delay24 : Delay  DelayLength=7  SampleTime=Ts
  Delay25 : Delay  DelayLength=8  SampleTime=Ts
  Delay26 : Delay  DelayLength=9  SampleTime=Ts
  Delay27 : Delay  DelayLength=10  SampleTime=Ts
  Delay30 : Delay  DelayLength=15  SampleTime=Ts
  Delay31 : Delay  DelayLength=16  SampleTime=Ts
  Delay32 : Delay  DelayLength=17  SampleTime=Ts
  Delay33 : Delay  DelayLength=18  SampleTime=Ts
  Delay34 : Delay  DelayLength=19  SampleTime=Ts
  Divide1 : Product  Inputs=*/
  Out1 : Outport
  wires:
  Delay31/1 -> Add9/17
  Delay30/1 -> Add9/16
  Delay14/1 -> Add9/2
  Add9/1 -> Divide1/1
  Delay17/1 -> Add9/12
  Delay19/1 -> Add9/14
  Delay23/1 -> Add9/7
  Delay25/1 -> Add9/9
  Delay26/1 -> Add9/10
  Delay18/1 -> Add9/13
  Delay24/1 -> Add9/8
  Delay20/1 -> Add9/4
  Delay21/1 -> Add9/5
  Delay15/1 -> Add9/3
  Delay32/1 -> Add9/18
  Delay34/1 -> Add9/20
  Delay33/1 -> Add9/19
  Delay22/1 -> Add9/6
  Constant2/1 -> Divide1/2
  Delay27/1 -> Add9/11
  In1/1 -> Delay14/1, Add9/1, Delay15/1, Delay20/1, Delay21/1, Delay34/1, Delay33/1, Delay32/1, Delay31/1, Delay30/1, Delay16/1, Delay19/1, Delay18/1, Delay17/1, Delay27/1, Delay26/1, Delay25/1, Delay24/1, Delay23/1, Delay22/1
  Delay16/1 -> Add9/15
  Divide1/1 -> Out1/1

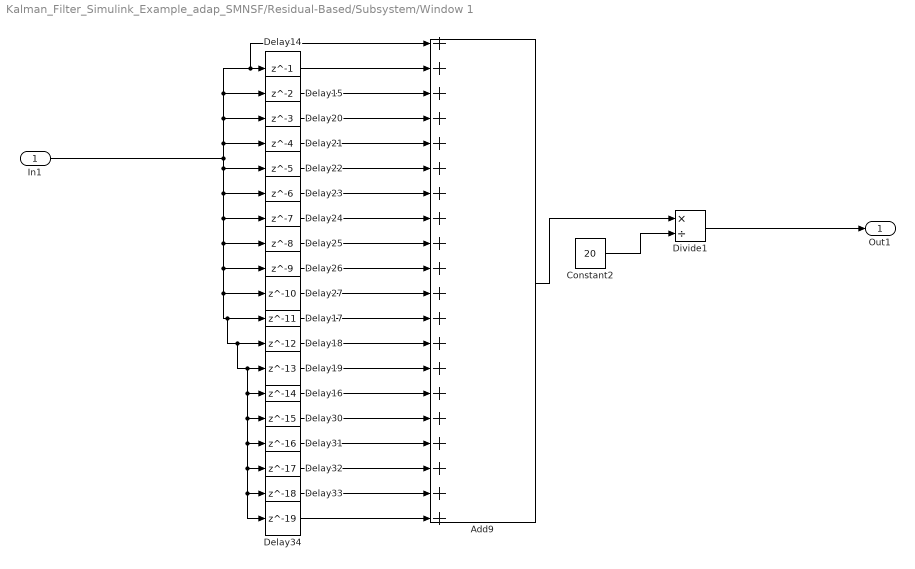
== system Kalman_Filter_Simulink_Example_adap_SMNSF/Residual-Based/Subsystem/Window 1 ==
  In1 : Inport
  Add9 : Sum  Inputs=20
  Constant2 : Constant  Value=20
  Delay14 : Delay  DelayLength=1  SampleTime=Ts
  Delay15 : Delay  SampleTime=Ts
  Delay16 : Delay  DelayLength=14  SampleTime=Ts
  Delay17 : Delay  DelayLength=11  SampleTime=Ts
  Delay18 : Delay  DelayLength=12  SampleTime=Ts
  Delay19 : Delay  DelayLength=13  SampleTime=Ts
  Delay20 : Delay  DelayLength=3  SampleTime=Ts
  Delay21 : Delay  DelayLength=4  SampleTime=Ts
  Delay22 : Delay  DelayLength=5  SampleTime=Ts
  Delay23 : Delay  DelayLength=6  SampleTime=Ts
  Delay24 : Delay  DelayLength=7  SampleTime=Ts
  Delay25 : Delay  DelayLength=8  SampleTime=Ts
  Delay26 : Delay  DelayLength=9  SampleTime=Ts
  Delay27 : Delay  DelayLength=10  SampleTime=Ts
  Delay30 : Delay  DelayLength=15  SampleTime=Ts
  Delay31 : Delay  DelayLength=16  SampleTime=Ts
  Delay32 : Delay  DelayLength=17  SampleTime=Ts
  Delay33 : Delay  DelayLength=18  SampleTime=Ts
  Delay34 : Delay  DelayLength=19  SampleTime=Ts
  Divide1 : Product  Inputs=*/
  Out1 : Outport
  wires:
  Delay31/1 -> Add9/17
  Delay30/1 -> Add9/16
  Delay14/1 -> Add9/2
  Add9/1 -> Divide1/1
  Delay17/1 -> Add9/12
  Delay19/1 -> Add9/14
  Delay23/1 -> Add9/7
  Delay25/1 -> Add9/9
  Delay26/1 -> Add9/10
  Delay18/1 -> Add9/13
  Delay24/1 -> Add9/8
  Delay20/1 -> Add9/4
  Delay21/1 -> Add9/5
  Delay15/1 -> Add9/3
  Delay32/1 -> Add9/18
  Delay34/1 -> Add9/20
  Delay33/1 -> Add9/19
  Delay22/1 -> Add9/6
  Constant2/1 -> Divide1/2
  Delay27/1 -> Add9/11
  In1/1 -> Delay14/1, Add9/1, Delay15/1, Delay20/1, Delay21/1, Delay34/1, Delay33/1, Delay32/1, Delay31/1, Delay30/1, Delay16/1, Delay19/1, Delay18/1, Delay17/1, Delay27/1, Delay26/1, Delay25/1, Delay24/1, Delay23/1, Delay22/1
  Delay16/1 -> Add9/15
  Divide1/1 -> Out1/1

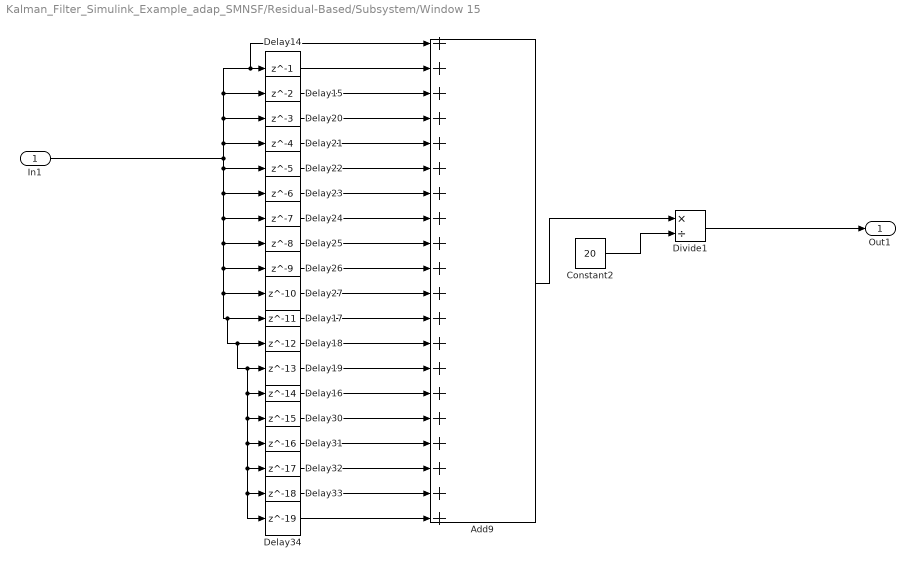
== system Kalman_Filter_Simulink_Example_adap_SMNSF/Residual-Based/Subsystem/Window 15 ==
  In1 : Inport
  Add9 : Sum  Inputs=20
  Constant2 : Constant  Value=20
  Delay14 : Delay  DelayLength=1  SampleTime=Ts
  Delay15 : Delay  SampleTime=Ts
  Delay16 : Delay  DelayLength=14  SampleTime=Ts
  Delay17 : Delay  DelayLength=11  SampleTime=Ts
  Delay18 : Delay  DelayLength=12  SampleTime=Ts
  Delay19 : Delay  DelayLength=13  SampleTime=Ts
  Delay20 : Delay  DelayLength=3  SampleTime=Ts
  Delay21 : Delay  DelayLength=4  SampleTime=Ts
  Delay22 : Delay  DelayLength=5  SampleTime=Ts
  Delay23 : Delay  DelayLength=6  SampleTime=Ts
  Delay24 : Delay  DelayLength=7  SampleTime=Ts
  Delay25 : Delay  DelayLength=8  SampleTime=Ts
  Delay26 : Delay  DelayLength=9  SampleTime=Ts
  Delay27 : Delay  DelayLength=10  SampleTime=Ts
  Delay30 : Delay  DelayLength=15  SampleTime=Ts
  Delay31 : Delay  DelayLength=16  SampleTime=Ts
  Delay32 : Delay  DelayLength=17  SampleTime=Ts
  Delay33 : Delay  DelayLength=18  SampleTime=Ts
  Delay34 : Delay  DelayLength=19  SampleTime=Ts
  Divide1 : Product  Inputs=*/
  Out1 : Outport
  wires:
  Delay31/1 -> Add9/17
  Delay30/1 -> Add9/16
  Delay14/1 -> Add9/2
  Add9/1 -> Divide1/1
  Delay17/1 -> Add9/12
  Delay19/1 -> Add9/14
  Delay23/1 -> Add9/7
  Delay25/1 -> Add9/9
  Delay26/1 -> Add9/10
  Delay18/1 -> Add9/13
  Delay24/1 -> Add9/8
  Delay20/1 -> Add9/4
  Delay21/1 -> Add9/5
  Delay15/1 -> Add9/3
  Delay32/1 -> Add9/18
  Delay34/1 -> Add9/20
  Delay33/1 -> Add9/19
  Delay22/1 -> Add9/6
  Constant2/1 -> Divide1/2
  Delay27/1 -> Add9/11
  In1/1 -> Delay14/1, Add9/1, Delay15/1, Delay20/1, Delay21/1, Delay34/1, Delay33/1, Delay32/1, Delay31/1, Delay30/1, Delay16/1, Delay19/1, Delay18/1, Delay17/1, Delay27/1, Delay26/1, Delay25/1, Delay24/1, Delay23/1, Delay22/1
  Delay16/1 -> Add9/15
  Divide1/1 -> Out1/1

== matlab function Kalman_Filter_Simulink_Example_adap_SMNSF/Residual-Based/Subsystem1/MATLAB Function ==
  data: x input; u input; y output
function y =Trans(x,u)

dt = 0.01;

y= x + [x(2); -9.81/0.5*sin(x(1))+u]*dt;
end

== matlab function Kalman_Filter_Simulink_Example_adap_SMNSF/Innovation-Based/Subsystem1/MATLAB Function ==
  data: x input; u input; y output
function y =Trans(x,u)

dt = 0.01;

y= x + [x(2); -9.81/0.5*sin(x(1))+u]*dt;
end
